simulink model "state_machine"  (R2016a)
settings: Solver=FixedStepDiscrete  StartTime=0.0  StopTime=100  FixedStep=0.01  MaxStep=0.01  RelTol=1e-3
undefined symbols (not defined in the file): track_1
libraries: lflib x7
settings Model: Creator=The MathWorks, Inc.  LastModifiedBy=bures
settings SolverCC: ZeroCrossAlgorithm=Adaptive
settings DataIOCC: LimitDataPoints=on
settings DebuggingCC: AllowSymbolicDim=off
settings ModelReferenceCC: PropagateSignalLabelsOutOfModel=off
settings GRTTargetCC: GeneratePreprocessorConditionals=Use local settings

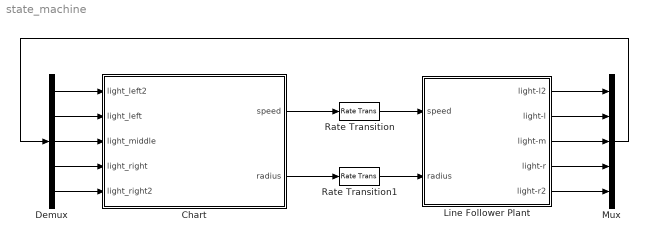
== system state_machine ==
  Chart : Stateflow chart  TreatAsAtomicUnit=on
  Demux : Demux  Outputs=5
  Line Follower Plant : Subsystem  mask{initX=506, initY=1050, initAngle=3/2*pi, trackCData=track_1, trackSamplesPerM=1000}
      mask prompts: initX "X (in mm)"; initY "Y (in mm)"; initAngle "Angle (in rad)"; trackCData "Track map"; trackSamplesPerM "Track map samples/m"
  Mux : Mux  Inputs=5
  Rate Transition : RateTransition  OutPortSampleTime=0.01
  Rate Transition1 : RateTransition  OutPortSampleTime=0.01
  wires:
  Chart/2(radius) -> Rate Transition1/1
  Chart/1(speed) -> Rate Transition/1
  Line Follower Plant/5(light-r2) -> Mux/5
  Line Follower Plant/4(light-r) -> Mux/4
  Line Follower Plant/3(light-m) -> Mux/3
  Line Follower Plant/2(light-l) -> Mux/2
  Line Follower Plant/1(light-l2) -> Mux/1
  Demux/1 -> Chart/1(light_left2)
  Demux/2 -> Chart/2(light_left)
  Demux/3 -> Chart/3(light_middle)
  Demux/4 -> Chart/4(light_right)
  Demux/5 -> Chart/5(light_right2)
  Mux/1 -> Demux/1
  Rate Transition/1 -> Line Follower Plant/1(speed)
  Rate Transition1/1 -> Line Follower Plant/2(radius)

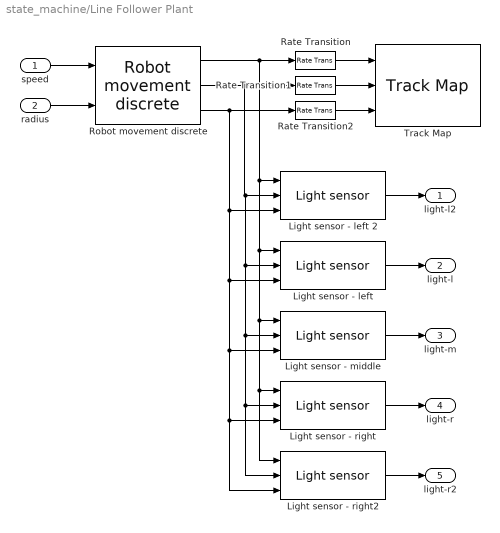
== system state_machine/Line Follower Plant ==
  speed : Inport
  radius : Inport  Port=2
  Light sensor - left : lflib/Light sensor  trackCData=trackCData  trackSamplesPerM=trackSamplesPerM  sensorPos=[150 30]
  Light sensor - left 2 : lflib/Light sensor  trackCData=trackCData  trackSamplesPerM=trackSamplesPerM  sensorPos=[150 70]
  Light sensor - middle : lflib/Light sensor  trackCData=trackCData  trackSamplesPerM=trackSamplesPerM  sensorPos=[150 0]
  Light sensor - right : lflib/Light sensor  trackCData=trackCData  trackSamplesPerM=trackSamplesPerM  sensorPos=[150 -30]
  Light sensor - right2 : lflib/Light sensor  trackCData=trackCData  trackSamplesPerM=trackSamplesPerM  sensorPos=[150 -70]
  Rate Transition : RateTransition
  Rate Transition1 : RateTransition
  Rate Transition2 : RateTransition
  Robot movement discrete : lflib/Robot movement discrete  initX=initX  initY=initY  initAngle=initAngle
  Track Map : lflib/Track Map  trackCData=trackCData  trackSamplesPerM=trackSamplesPerM
  light-l2 : Outport
  light-l : Outport  Port=2
  light-m : Outport  Port=3
  light-r : Outport  Port=4
  light-r2 : Outport  Port=5
  wires:
  Light sensor - right2/1 -> light-r2/1
  Light sensor - left/1 -> light-l/1
  Light sensor - middle/1 -> light-m/1
  Light sensor - left 2/1 -> light-l2/1
  Light sensor - right/1 -> light-r/1
  Robot movement discrete/1 -> Light sensor - right2/1, Light sensor - right/1, Light sensor - middle/1, Light sensor - left/1, Light sensor - left 2/1, Rate Transition/1
  Robot movement discrete/2 -> Light sensor - right2/2, Light sensor - right/2, Light sensor - middle/2, Light sensor - left/2, Light sensor - left 2/2, Rate Transition1/1
  radius/1 -> Robot movement discrete/2
  speed/1 -> Robot movement discrete/1
  Robot movement discrete/3 -> Light sensor - left/3, Light sensor - middle/3, Light sensor - right/3, Light sensor - right2/3, Light sensor - left 2/3, Rate Transition2/1
  Rate Transition/1 -> Track Map/1
  Rate Transition1/1 -> Track Map/2
  Rate Transition2/1 -> Track Map/3

== stateflow chart state_machine/Chart ==
  state Lap_state [parallel]
    settings: executionOrder=1
    state Init
    state Looking_for_start
    state Start_found
    state Started
    state Beyond_start_line
    (default) -> Init
    Init -> Looking_for_start : /{send(start)}
    Looking_for_start -> Start_found : [light_left2 < 0.5]/{send(stop)}
    Start_found -> Started : after(1,sec)/{send(start)}
    Started -> Beyond_start_line : [light_left2 > 0.5]
  state Driving_state [parallel]
    settings: executionOrder=2
    state Driving
      state Straight
        du:
        speed=100;
        radius=0;
      state Right
        du:
        speed=100;
        radius=100;
      state Left
        du:
        speed=100;
        radius=-100;
      (default) -> Straight
      Straight -> Right [order 1] : [light_middle < 0.5]
      Right -> Straight : [light_middle > 0.5]
      Left -> Straight : [light_right > 0.5]
      Straight -> Left [order 2] : [light_right < 0.5]
    state Still
      du:
      speed=0;
      radius=0;
    Driving -> Still : stop
    Still -> Driving : start
    (default) -> Still
  data: light_left2 input; light_left input; light_middle input; light_right input; light_right2 input; speed output; radius output
  events: start local FUNCTION_CALL_EVENT; stop local FUNCTION_CALL_EVENT
